simulink model "SO_lQR"  (R2022a)
settings: Solver=VariableStepAuto  StartTime=0.0  StopTime=4  RelTol=1e-3
values from neighbouring files (symbols this model uses):
  K = lqr(A,B,Q,R)    [SO_LQR.m]
undefined symbols (not defined in the file or in its folder): speed
libraries: Solver_SF x1
settings Model: SimulationMode=accelerator  Creator=12567  LastModifiedBy=12567
settings DataIOCC: ReturnWorkspaceOutputs=off

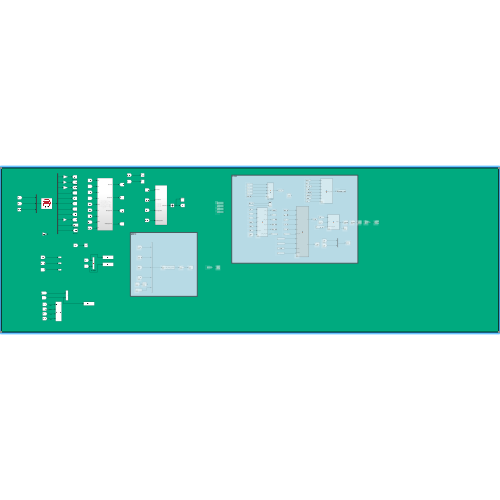
[thumbnail: Simulink's stored preview of the top-level diagram]
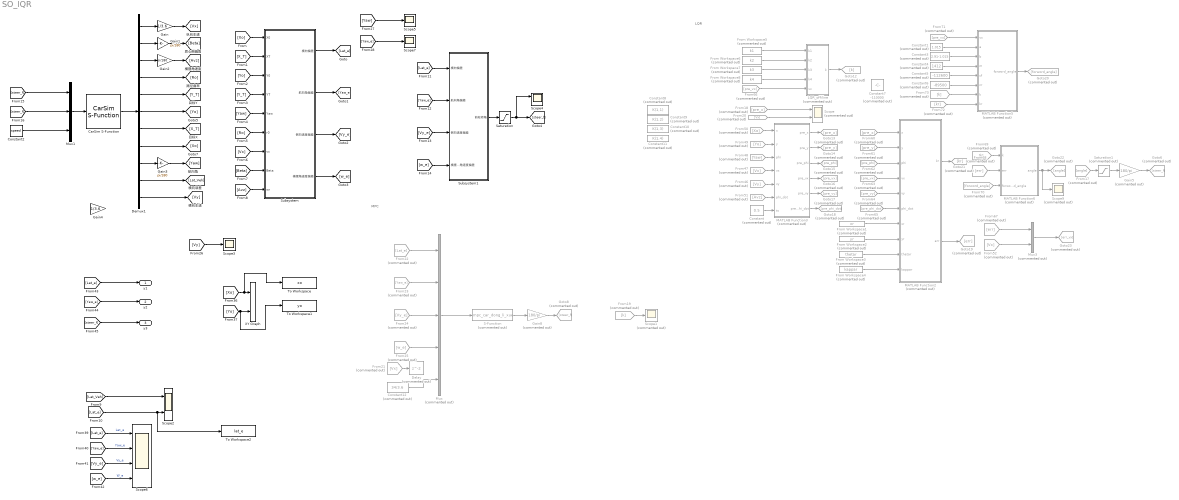
== system SO_lQR ==
  note: MPC
  note: LQR
  CarSim S-Function : Solver_SF/CarSim S-Function  Priority=1  SIMFILE=simfile.sim
  Constant : Constant  Commented=on  Value=0.5
  Constant1 : Constant  Commented=on  Value=1.015
  Constant10 : Constant  Commented=on  Value=K(1,3)
  Constant11 : Constant  Commented=on  Value=K(1,4)
  Constant12 : Constant  Commented=on  Value=34/3.6
  Constant2 : Constant  Value=speed
  Constant3 : Constant  Commented=on  Value=2.91-1.015
  Constant4 : Constant  Commented=on  Value=1412
  Constant5 : Constant  Commented=on  Value=-112600
  Constant6 : Constant  Commented=on  Value=-89500
  Constant7 : Constant  Commented=on  Value=-110000
  Constant8 : Constant  Commented=on  Value=K(1,1)
  Constant9 : Constant  Commented=on  Value=K(1,2)
  Delay : Delay  Commented=on
  Demux1 : Demux  Outputs=11
  From Workspace1 : FromWorkspace  Commented=on  VariableName=xr
  From Workspace2 : FromWorkspace  Commented=on  VariableName=yr
  From Workspace3 : FromWorkspace  Commented=on  VariableName=thetar
  From Workspace4 : FromWorkspace  Commented=on  VariableName=kappar
  From Workspace5 : FromWorkspace  Commented=on  VariableName=k1
  From Workspace6 : FromWorkspace  Commented=on  VariableName=k2
  From Workspace7 : FromWorkspace  Commented=on  VariableName=k3
  From Workspace8 : FromWorkspace  Commented=on  VariableName=k4
  From17 : From  Commented=on  GotoTag=angle
  From18 : From  Commented=on  GotoTag=pre_x
  From19 : From  Commented=on  GotoTag=k
  From{20..21,47,52} (4 alike) : From  Commented=on  GotoTag=Vx
  From22 : From  Commented=on  GotoTag=Lat_e
  From23 : From  Commented=on  GotoTag=Yaw_e
  From24 : From  Commented=on  GotoTag=Vy_e
  From25 : From  Commented=on  GotoTag=w_e
  From46 : From  Commented=on  GotoTag=Vy
  From48 : From  Commented=on  GotoTag=Yaw
  From49 : From  Commented=on  GotoTag=Yo
  From50 : From  Commented=on  GotoTag=Xo
  From51 : From  Commented=on  GotoTag=Avz
  From60 : From  Commented=on  GotoTag=pre_x
  From61 : From  Commented=on  GotoTag=pre_y
  From62 : From  Commented=on  GotoTag=pre_phi
  From63 : From  Commented=on  GotoTag=pre_vx
  From64 : From  Commented=on  GotoTag=pre_vy
  From65 : From  Commented=on  GotoTag=pre_phi_dot
  From66 : From  Commented=on  GotoTag=pre_vx
  From67 : From  Commented=on  GotoTag=err
  From68 : From  Commented=on  GotoTag=err
  From69 : From  Commented=on  GotoTag=k
  From70 : From  Commented=on  GotoTag=forword_angle
  From71 : From  Commented=on  GotoTag=pre_vx
  From72 : From  Commented=on  GotoTag=kr
  From73 : From  Commented=on  GotoTag=k
  Gain : Gain  Gain=1/3.6
  Gain1 : Gain  Gain=pi/180
  Gain2 : Gain  Gain=pi/180
  Gain3 : Gain  Gain=pi/180
  Gain4 : Gain  Gain=1/3.6
  Gain5 : Gain  Commented=on  Gain=180/pi
  Gain8 : Gain  Commented=on  Gain=180/pi
  Goto12 : Goto  Commented=on  GotoTag=k
  Goto13 : Goto  Commented=on  GotoTag=pre_x
  Goto14 : Goto  Commented=on  GotoTag=pre_y
  Goto15 : Goto  Commented=on  GotoTag=pre_phi
  Goto16 : Goto  Commented=on  GotoTag=pre_vx
  Goto17 : Goto  Commented=on  GotoTag=pre_vy
  Goto18 : Goto  Commented=on  GotoTag=pre_phi_dot
  Goto19 : Goto  Commented=on  GotoTag=err
  Goto20 : Goto  Commented=on  GotoTag=forword_angle
  Goto21 : Goto  Commented=on  GotoTag=kr
  Goto22 : Goto  Commented=on  GotoTag=angle
  Goto23 : Goto  Commented=on  GotoTag=err_vx
  Goto6 : Goto  Commented=on  GotoTag=steer_f
  Goto8 : Goto  Commented=on  GotoTag=steer_f
  LQR_offiline : MATLAB Function  Commented=on  TreatAsAtomicUnit=on
  MATLAB Function2 : MATLAB Function  Commented=on  TreatAsAtomicUnit=on
  MATLAB Function3 : MATLAB Function  Commented=on  TreatAsAtomicUnit=on
  MATLAB Function5 : MATLAB Function  Commented=on  TreatAsAtomicUnit=on
  MATLAB Function6 : MATLAB Function  Commented=on  TreatAsAtomicUnit=on
  Mux : Mux  Commented=on  Inputs=5
  Mux1 : Mux  Inputs=3
  Mux3 : Mux  Commented=on  Inputs=2
  S-Function : S-Function  Commented=on  FunctionName=mpc_car_dong_li_xue  SFunctionDeploymentMode=off  EnableBusSupport=off
  Saturation : Saturate  UpperLimit=30  LowerLimit=-30
  Saturation1 : Saturate  Commented=on  UpperLimit=40  LowerLimit=-40
  Scope : Scope  Commented=on  NumInputPorts=2
  Scope1 : Scope  Commented=on
  Scope2 : Scope  NumInputPorts=2
  Scope3 : Scope
  Scope4 : Scope  NumInputPorts=2
  Scope5 : Scope
  Scope6 : Scope  NumInputPorts=4
  Scope7 : Scope
  Scope9 : Scope  Commented=on
  Subsystem : Subsystem
  Subsystem1 : Subsystem
  To Workspace : ToWorkspace  VariableName=xo  SampleTime=-1
      settings: Save2DSignal=2-D array (concatenate along first dimension)
  To Workspace1 : ToWorkspace  VariableName=yo  SampleTime=-1
      settings: Save2DSignal=2-D array (concatenate along first dimension)
  To Workspace2 : ToWorkspace  VariableName=lat_e  SampleTime=-1
      settings: Save2DSignal=2-D array (concatenate along first dimension)
  XY Graph : Record  FileSettingsInternal="{\"entries\":[{\"content\":{\"excelSettings\":{\"content\":{},\"type\":\"Streamout.ExcelSettings\"}},\"type\":\"Streamout.FileSettingStorage\",\"uuid\":\"\"}],\"packageUris\":[\"http:\\/\\/schema.mathworks.com\\/mf0\\/streamout_blocks\\/R2020a\"],\"version\":\"1.0\"}"  Layout=[1 1]  SignalsInternal="{\"entries\":[{\"content\":{\"signals\":[{\"content\":{\"blockPath\":[],\"channel\":[],\"dimensions\":[1],\"domain\":\"\",\"lineColor\":\"#fe330a\",\"plots\":[],\"port\":1,\"sid\":[\"\"],\"signalID\":1067719,\"signalName\":\"From36\"},\"type\":\"RecordBlkView.Signal\",\"uuid\":\"\"},{\"content\":{\"blockPath\":[],\"channel\":[],\"dimensions\":[1],\"domain\":\"\",\"lineColor\":\"#22b573\",\"plots\":[],\"port\":2,\"sid\":[\"\"],\"signalID\":1067723,\"signalName\":\"From37\"},\"type\":\"RecordBlkView.Signal\",\"uuid\":\"\"}]},\"type\":\"RecordBlkView.InputSignals\",\"uuid\":\"\"}],\"packageUris\":[\"http:\\/\\/schema.mathworks.com\\/mf0\\/streamout_blocks\\/R2020a\"],\"version\":\"1.0\"}"  VisualizationBindings="{\"xyplotplugin\":{\"info\":[{\"series\":[],\"subplotID\":1}]}}"  CompatibilityTag=XY
  y1 : Outport
  y2 : Outport  Port=2
  y3 : Outport  Port=3
  wires:
  CarSim S-Function/1 -> Demux1/1
  Gain1/1 -> [Beta]
  Demux1/1 -> Gain/1
  Demux1/3 -> Gain2/1
  Demux1/5 -> [Y_T]
  Demux1/10 -> [Lat_Veh]
  Demux1/4 -> [Ro]
  Gain3/1 -> [Yaw]
  Demux1/7 -> [X_T]
  Demux1/9 -> Gain3/1
  Gain2/1 -> [Avz]
  Demux1/6 -> [Yo]
  Demux1/2 -> Gain1/1
  Demux1/8 -> [Xo]
  Gain/1 -> [Vx]
  Subsystem/1(横向偏差) -> [Lat_e]
  [Avz] -> Subsystem/9(wr)
  Subsystem/2(航向角偏差) -> [Yaw_e]
  [Ro] -> Subsystem/6(r0)
  [Xo] -> Subsystem/1(X0)
  Subsystem/3(侧向速度偏差) -> [Vy_e]
  [Vx] -> Subsystem/7(vx)
  [Y_T] -> Subsystem/4(YT)
  Subsystem/4(横摆角速度偏差) -> [w_e]
  [Yaw] -> Subsystem/5(Yaw)
  [Beta] -> Subsystem/8(Beta)
  [X_T] -> Subsystem/2(XT)
  [Yo] -> Subsystem/3(Y0)
  [Yo] -> To Workspace1/1, XY Graph/2
  [steer_f] -> y3/1
  [Lat_e] -> y1/1
  [w_e] -> Subsystem1/4(横摆角速度偏差)
  [Lat_e] -> Subsystem1/1(横向偏差)
  [Vy_e] -> Subsystem1/3(侧向速度偏差)
  [Yaw_e] -> y2/1
  [Xo] -> To Workspace/1, XY Graph/1
  Subsystem1/1(前轮转角) -> Saturation/1
  Saturation/1 -> Scope4/1, [steer_f]
  [Yaw_e] -> Subsystem1/2(航向角偏差)
  [w_e] -> Scope6/4  "W_e"
  [Vy_e] -> Scope6/3  "Vy_e"
  [Lat_e] -> To Workspace2/1, Scope2/2
  [Lat_e] -> Scope6/1  "Lat_e"
  [Lat_Veh] -> Scope2/1
  [Yaw_e] -> Scope6/2  "Yaw_e"
  [steer_f] -> Mux1/1
  [steer_f] -> Mux1/2
  Mux1/1 -> CarSim S-Function/1
  MATLAB Function2/1(kr) -> Goto21/1
  Constant5/1 -> MATLAB Function5/5(cf)
  MATLAB Function3/4(pre_vx) -> Goto16/1
  From60/1 -> MATLAB Function2/1(x)
  Constant6/1 -> MATLAB Function5/6(cr)
  From50/1 -> MATLAB Function3/1(x)
  From47/1 -> MATLAB Function3/4(vx)
  From49/1 -> MATLAB Function3/2(y)
  LQR_offiline/1(k) -> Goto12/1
  From48/1 -> MATLAB Function3/3(phi)
  From72/1 -> MATLAB Function5/8(kr)
  Mux3/1 -> Goto23/1
  From65/1 -> MATLAB Function2/6(phi_dot)
  From64/1 -> MATLAB Function2/5(vy)
  Constant3/1 -> MATLAB Function5/3(b)
  MATLAB Function6/1(angle) -> Scope9/1, Goto22/1
  From62/1 -> MATLAB Function2/3(phi)
  From61/1 -> MATLAB Function2/2(y)
  From70/1 -> MATLAB Function6/3(forword_angle)
  From68/1 -> MATLAB Function6/2(err)
  Constant1/1 -> MATLAB Function5/2(a)
  From67/1 -> Mux3/1
  From66/1 -> LQR_offiline/5(vx)
  MATLAB Function2/2(err) -> Goto19/1
  From63/1 -> MATLAB Function2/4(vx)
  Constant4/1 -> MATLAB Function5/4(m)
  MATLAB Function3/6(pre_phi_dot) -> Goto18/1
  From71/1 -> MATLAB Function5/1(vx)
  MATLAB Function5/1(forword_angle) -> Goto20/1
  From69/1 -> MATLAB Function6/1(k)
  Constant/1 -> MATLAB Function3/7(ts)
  From46/1 -> MATLAB Function3/5(vy)
  From51/1 -> MATLAB Function3/6(phi_dot)
  MATLAB Function3/5(pre_vy) -> Goto17/1
  MATLAB Function3/2(pre_y) -> Goto14/1
  From Workspace3/1 -> MATLAB Function2/9(thetar)
  MATLAB Function3/3(pre_phi) -> Goto15/1
  From73/1 -> MATLAB Function5/7(k)
  From52/1 -> Mux3/2
  From Workspace4/1 -> MATLAB Function2/10(kappar)
  MATLAB Function3/1(pre_x) -> Goto13/1
  Gain5/1 -> Goto6/1
  Saturation1/1 -> Gain5/1
  From17/1 -> Saturation1/1
  From Workspace1/1 -> MATLAB Function2/7(xr)
  From Workspace2/1 -> MATLAB Function2/8(yr)
  From18/1 -> Scope/1
  From19/1 -> Scope1/1
  From20/1 -> Scope/2
  From24/1 -> Mux/3
  S-Function/1 -> Gain8/1
  Mux/1 -> S-Function/1
  From22/1 -> Mux/1
  From23/1 -> Mux/2
  From25/1 -> Mux/4
  Gain8/1 -> Goto8/1
  From21/1 -> Delay/1
  Constant12/1 -> Mux/5
  From Workspace5/1 -> LQR_offiline/1(k1)
  From Workspace6/1 -> LQR_offiline/2(k2)
  From Workspace7/1 -> LQR_offiline/3(k3)
  From Workspace8/1 -> LQR_offiline/4(k4)
  Demux1/11 -> [Vy]
  [Vy] -> Scope3/1
  Constant2/1 -> Mux1/3
  [Yaw] -> Scope5/1
  [Yaw_e] -> Scope7/1

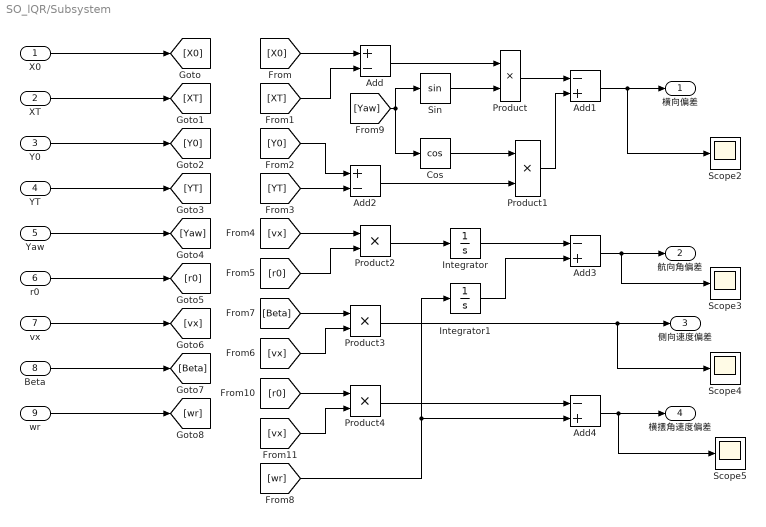
== system SO_lQR/Subsystem ==
  X0 : Inport
  XT : Inport  Port=2
  Y0 : Inport  Port=3
  YT : Inport  Port=4
  Yaw : Inport  Port=5
  r0 : Inport  Port=6
  vx : Inport  Port=7
  Beta : Inport  Port=8
  wr : Inport  Port=9
  Add : Sum  Inputs=+-
  Add1 : Sum  Inputs=-+
  Add2 : Sum  Inputs=+-
  Add3 : Sum  Inputs=-+
  Add4 : Sum  Inputs=-+
  Cos : Trigonometry  Operator=cos
  Integrator : Integrator
  Integrator1 : Integrator
  Product{,1..4} (5 alike) : Product
  Scope{2..5} (4 alike) : Scope
  Sin : Trigonometry
  横向偏差 : Outport
  航向角偏差 : Outport  Port=2
  侧向速度偏差 : Outport  Port=3
  横摆角速度偏差 : Outport  Port=4
  wires:
  Add4/1 -> 横摆角速度偏差/1, Scope5/1
  Product2/1 -> Integrator/1
  [vx] -> Product4/2
  Beta/1 -> [Beta]
  wr/1 -> [wr]
  Product3/1 -> 侧向速度偏差/1, Scope4/1
  [Yaw] -> Cos/1, Sin/1
  [Y0] -> Add2/1
  [vx] -> Product2/1
  Integrator1/1 -> Add3/2
  Add1/1 -> 横向偏差/1, Scope2/1
  Add3/1 -> 航向角偏差/1, Scope3/1
  Product1/1 -> Add1/2
  [YT] -> Add2/2
  XT/1 -> [XT]
  r0/1 -> [r0]
  [Beta] -> Product3/1
  X0/1 -> [X0]
  Y0/1 -> [Y0]
  YT/1 -> [YT]
  Cos/1 -> Product1/1
  Yaw/1 -> [Yaw]
  Integrator/1 -> Add3/1
  Add/1 -> Product/1
  [X0] -> Add/1
  [wr] -> Integrator1/1, Add4/2
  vx/1 -> [vx]
  [vx] -> Product3/2
  Add2/1 -> Product1/2
  [r0] -> Product4/1
  [XT] -> Add/2
  Product4/1 -> Add4/1
  Product/1 -> Add1/1
  Sin/1 -> Product/2
  [r0] -> Product2/2

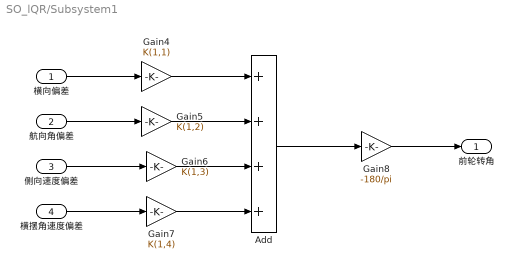
== system SO_lQR/Subsystem1 ==
  横向偏差 : Inport
  航向角偏差 : Inport  Port=2
  侧向速度偏差 : Inport  Port=3
  横摆角速度偏差 : Inport  Port=4
  Add : Sum  Inputs=++++
  Gain4 : Gain  Gain=K(1,1)
  Gain5 : Gain  Gain=K(1,2)
  Gain6 : Gain  Gain=K(1,3)
  Gain7 : Gain  Gain=K(1,4)
  Gain8 : Gain  Gain=-180/pi
  前轮转角 : Outport
  wires:
  Gain4/1 -> Add/1
  Gain7/1 -> Add/4
  Gain5/1 -> Add/2
  Add/1 -> Gain8/1
  侧向速度偏差/1 -> Gain6/1
  Gain6/1 -> Add/3
  横摆角速度偏差/1 -> Gain7/1
  横向偏差/1 -> Gain4/1
  航向角偏差/1 -> Gain5/1
  Gain8/1 -> 前轮转角/1

== matlab function SO_lQR/MATLAB Function2 ==
  data: x input; kr output; y input; phi input; vx input; vy input; phi_dot input; xr input; yr input; thetar input; kappar input; err output
function [kr,err] = fcn(x,y,phi,vx,vy,phi_dot,xr,yr,thetar,kappar)
    n=length(xr);
    d_min=(x-xr(1))^2+(y-yr(1))^2;
    min=1;
    for i=1:n
        d=(x-xr(i))^2+(y-yr(i))^2;
        if d<d_min
            d_min=d;
            min=i;
        end
    end
    dmin=min;
    tor=[cos(thetar(dmin));sin(thetar(dmin))];
    nor=[-sin(thetar(dmin));cos(thetar(dmin))];
    d_err=[x-xr(dmin);y-yr(dmin)];
    ed=nor'*d_err;
    es=tor'*d_err;
    %projection_point_thetar=thetar(dmin);%apollo
    projection_point_thetar=thetar(dmin)+kappar(dmin)*es;
    ed_dot=vy*cos(phi-projection_point_thetar)+vx*sin(phi-projection_point_thetar);
    %%%%%%%%%
    ephi=sin(phi-projection_point_thetar);
    %%%%%%%%%
    s_dot=vx*cos(phi-projection_point_thetar)-vy*sin(phi-projection_point_thetar);
    s_dot=s_dot/(1-kappar(dmin)*ed);
    ephi_dot=phi_dot-kappar(dmin)*s_dot;
    kr=kappar(dmin);
    err=[ed;ed_dot;ephi;ephi_dot];%lqr
%  err=[ed;ephi;ed_dot;ephi_dot];   %mpc
end

== matlab function SO_lQR/MATLAB Function3 ==
  data: x input; pre_x output; y input; phi input; vx input; vy input; phi_dot input; ts input; pre_y output; pre_phi output; pre_vx output; pre_vy output; pre_phi_dot output
function [pre_x,pre_y,pre_phi,pre_vx,pre_vy,pre_phi_dot] = fcn(x,y,phi,vx,vy,phi_dot,ts)
    pre_x=x+vx*ts*cos(phi)-vy*ts*sin(phi);
    pre_y=y+vy*ts*cos(phi)+vx*ts*sin(phi);
    pre_phi=phi+phi_dot*ts;
    pre_vx=vx;
    pre_vy=vy;
    pre_phi_dot=phi_dot;
end

== matlab function SO_lQR/LQR_offiline ==
  data: k1 input; k output; k2 input; k3 input; k4 input; vx input
function k  = fcn(k1,k2,k3,k4,vx)
    if abs(vx)<0.01
        k=[0,0,0,0];
    else
        index=round(vx/0.01);
        k=[k1(index),k2(index),k3(index),k4(index)];
%  k=[k1,k2,k3,k4];
    end
end

== matlab function SO_lQR/MATLAB Function5 ==
  data: vx input; forword_angle output; a input; b input; m input; cf input; cr input; k input; kr input
function forword_angle = fcn(vx,a,b,m,cf,cr,k,kr)
    forword_angle=kr*(a+b-b*k(3)-(m*vx*vx/(a+b))*((b/cf)+(a/cr)*k(3)-(a/cr)));
end

== matlab function SO_lQR/MATLAB Function6 ==
  data: k input; angle output; err input; forword_angle input
function angle = fcn(k,err,forword_angle)

    angle=-k*err+forword_angle;
end
